simulink model "mdl3"  (R2022b)
settings: Solver=VariableStepAuto  StartTime=0.0  StopTime=3000  RelTol=1e-3
undefined symbols (not defined in the file or in its folder): DiscIntNeverNeededParam
libraries: simulink x7, rllib x1
settings Model: Creator=yonat  LastModifiedBy=yonat

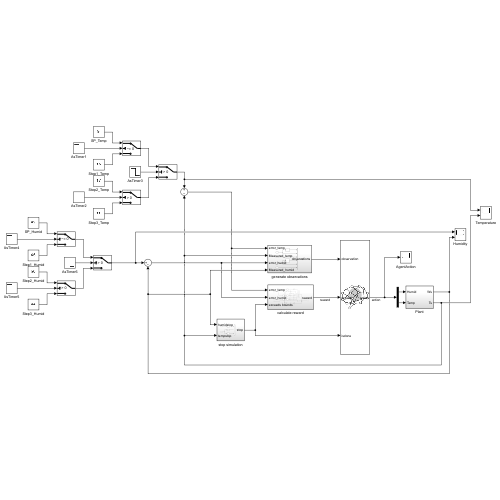
[thumbnail: Simulink's stored preview of the top-level diagram]
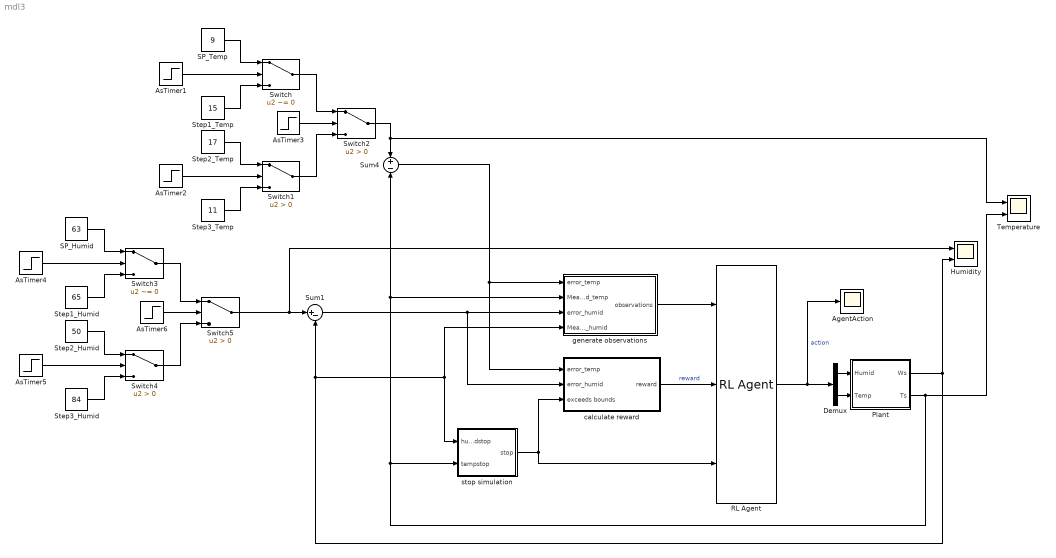
== system mdl3 ==
  AgentAction : Scope
  AsTimer1 : Step  Time=600  Before=1  After=0  SampleTime=0
  AsTimer2 : Step  Time=1800  Before=1  After=0  SampleTime=0
  AsTimer3 : Step  Time=1200  Before=1  After=0  SampleTime=0
  AsTimer4 : Step  Time=600  Before=1  After=0  SampleTime=0
  AsTimer5 : Step  Time=1800  Before=1  After=0  SampleTime=0
  AsTimer6 : Step  Time=1200  Before=1  After=0  SampleTime=0
  Demux : Demux  Outputs=2
  Humidity : Scope  NumInputPorts=2
  Plant : Subsystem
  RL Agent : rllib/RL Agent  Agent=agentObj  ExternalActionAsInput=off  ProvideLastAction=off  ProvideCumRwd=off  TreatAsDirectFeedthrough=on  UseStrictObservationDataTypes=off
  SP_Humid : Constant  Value=63
  SP_Temp : Constant  Value=9
  Step1_Humid : Constant  Value=65
  Step1_Temp : Constant  Value=15
  Step2_Humid : Constant  Value=50
  Step2_Temp : Constant  Value=17
  Step3_Humid : Constant  Value=84
  Step3_Temp : Constant  Value=11
  Sum1 : Sum  Inputs=|+-  SaturateOnIntegerOverflow=on
  Sum4 : Sum  Inputs=+-  SaturateOnIntegerOverflow=on
  Switch : Switch  Criteria=u2 ~= 0  Threshold=1  SaturateOnIntegerOverflow=off  InputSameDT=off
  Switch{1..2,4..5} (4 alike) : Switch  Criteria=u2 > Threshold  SaturateOnIntegerOverflow=off  InputSameDT=off
  Switch3 : Switch  Criteria=u2 ~= 0  Threshold=1  SaturateOnIntegerOverflow=off  InputSameDT=off
  Temperature : Scope  NumInputPorts=2
  calculate reward : Subsystem
  generate observations : Subsystem
  stop simulation : Subsystem
  wires:
  stop simulation/1(stop) -> calculate reward/3(exceeds bounds), RL Agent/3
  Plant/2(Ts) -> generate observations/2(Measured_temp), Sum4/2, stop simulation/2(tempstop), Temperature/2
  Sum4/1 -> generate observations/1(error_temp), calculate reward/1(error_temp)
  calculate reward/1(reward) -> RL Agent/2  "reward"
  Plant/1(Ws) -> generate observations/4(Measured_humid), stop simulation/1(humidstop), Sum1/2, Humidity/2
  Sum1/1 -> calculate reward/2(error_humid), generate observations/3(error_humid)
  RL Agent/1 -> AgentAction/1, Demux/1  "action"
  generate observations/1(observations) -> RL Agent/1
  Demux/2 -> Plant/2(Temp)
  Demux/1 -> Plant/1(Humid)
  SP_Temp/1 -> Switch/1
  AsTimer1/1 -> Switch/2
  Step3_Temp/1 -> Switch1/3
  Step1_Temp/1 -> Switch/3
  Switch/1 -> Switch2/1
  Switch1/1 -> Switch2/3
  AsTimer3/1 -> Switch2/2
  Step2_Temp/1 -> Switch1/1
  AsTimer2/1 -> Switch1/2
  Switch2/1 -> Temperature/1, Sum4/1
  AsTimer6/1 -> Switch5/2
  Step2_Humid/1 -> Switch4/1
  AsTimer5/1 -> Switch4/2
  Switch4/1 -> Switch5/3
  Step3_Humid/1 -> Switch4/3
  AsTimer4/1 -> Switch3/2
  Switch3/1 -> Switch5/1
  Step1_Humid/1 -> Switch3/3
  SP_Humid/1 -> Switch3/1
  Switch5/1 -> Humidity/1, Sum1/1

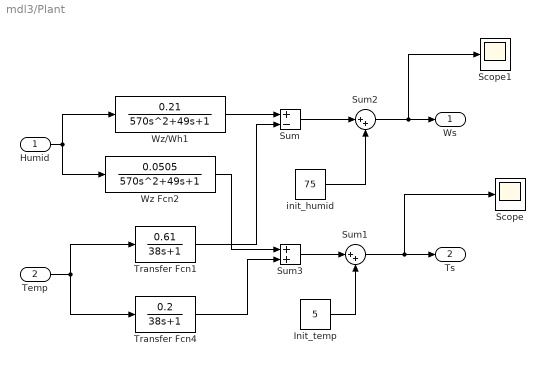
== system mdl3/Plant ==
  Humid : Inport
  Temp : Inport  Port=2
  Init_temp : Constant  Value=5
  Scope : Scope
  Scope1 : Scope
  Sum : Sum  Inputs=+-
  Sum1 : Sum  Inputs=|++
  Sum2 : Sum  Inputs=|++
  Sum3 : Sum
  Transfer Fcn1 : TransferFcn  Numerator=[0.61]  Denominator=[38 1]
  Transfer Fcn4 : TransferFcn  Numerator=[0.2]  Denominator=[38 1]
  Wz Fcn2 : TransferFcn  Numerator=[0.0505]  Denominator=[570 49 1]
  Wz/Wh1 : TransferFcn  Numerator=[0.21]  Denominator=[570 49 1]
  init_humid : Constant  Value=75
  Ws : Outport
  Ts : Outport  Port=2
  wires:
  Wz Fcn2/1 -> Sum3/1
  Humid/1 -> Wz/Wh1/1, Wz Fcn2/1
  Temp/1 -> Transfer Fcn1/1, Transfer Fcn4/1
  Transfer Fcn1/1 -> Sum/2
  Wz/Wh1/1 -> Sum/1
  Transfer Fcn4/1 -> Sum3/2
  Sum/1 -> Sum2/1
  Sum3/1 -> Sum1/1
  Sum1/1 -> Scope/1, Ts/1
  Sum2/1 -> Scope1/1, Ws/1
  Init_temp/1 -> Sum1/2
  init_humid/1 -> Sum2/2

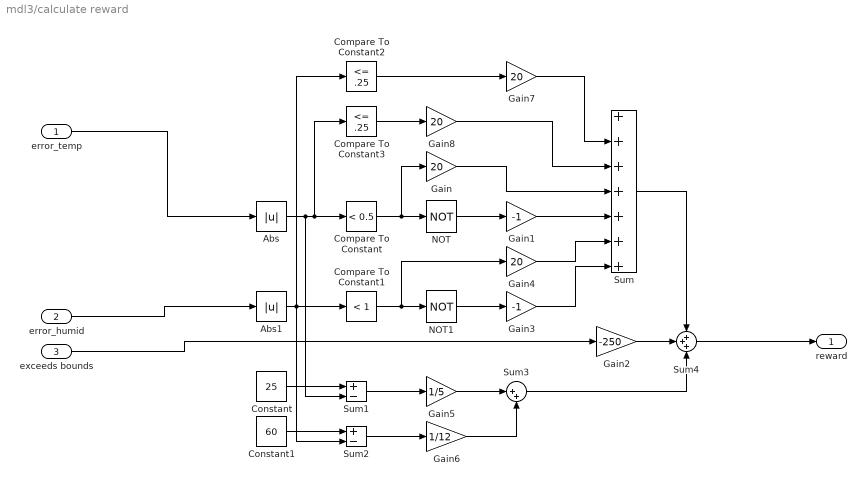
== system mdl3/calculate reward ==
  error_temp : Inport
  error_humid : Inport  Port=2
  exceeds bounds : Inport  Port=3
  Abs : Abs  SaturateOnIntegerOverflow=off
  Abs1 : Abs  SaturateOnIntegerOverflow=off
  Compare To Constant : simulink/Logic and Bit Operations/Compare To Constant  relop=<  const=0.5  OutDataTypeStr=boolean
  Compare To Constant1 : simulink/Logic and Bit Operations/Compare To Constant  relop=<  const=1  OutDataTypeStr=boolean
  Compare To Constant2 : simulink/Logic and Bit Operations/Compare To Constant  relop=<=  const=.25  OutDataTypeStr=boolean
  Compare To Constant3 : simulink/Logic and Bit Operations/Compare To Constant  relop=<=  const=.25  OutDataTypeStr=boolean
  Constant : Constant  Value=25
  Constant1 : Constant  Value=60
  Gain{,4,7..8} (4 alike) : Gain  Gain=20
  Gain1 : Gain  Gain=-1
  Gain2 : Gain  Gain=-250
  Gain3 : Gain  Gain=-1
  Gain5 : Gain  Gain=1/5
  Gain6 : Gain  Gain=1/12
  NOT : Logic  Operator=NOT  IconShape=distinctive  AllPortsSameDT=off  OutDataTypeStr=boolean
  NOT1 : Logic  Operator=NOT  IconShape=distinctive  AllPortsSameDT=off  OutDataTypeStr=boolean
  Sum : Sum  Inputs=+++++++  OutDataTypeStr=double
  Sum1 : Sum  Inputs=+-
  Sum2 : Sum  Inputs=+-
  Sum3 : Sum  Inputs=|++
  Sum4 : Sum  Inputs=+++
  reward : Outport  VectorParamsAs1DForOutWhenUnconnected=off
  wires:
  Compare To Constant2/1 -> Gain7/1
  Abs1/1 -> Compare To Constant1/1, Compare To Constant2/1, Sum2/2
  Sum3/1 -> Sum4/3
  NOT/1 -> Gain1/1
  Sum4/1 -> reward/1
  Gain7/1 -> Sum/2
  NOT1/1 -> Gain3/1
  Gain6/1 -> Sum3/2
  Sum2/1 -> Gain6/1
  Sum1/1 -> Gain5/1
  exceeds bounds/1 -> Gain2/1
  Compare To Constant1/1 -> Gain4/1, NOT1/1
  Gain/1 -> Sum/4
  Constant/1 -> Sum1/1
  Gain5/1 -> Sum3/1
  error_temp/1 -> Abs/1
  Compare To Constant/1 -> NOT/1, Gain/1
  Abs/1 -> Compare To Constant3/1, Compare To Constant/1, Sum1/2
  Sum/1 -> Sum4/1
  Gain2/1 -> Sum4/2
  Gain8/1 -> Sum/3
  Gain3/1 -> Sum/7
  Compare To Constant3/1 -> Gain8/1
  error_humid/1 -> Abs1/1
  Gain1/1 -> Sum/5
  Gain4/1 -> Sum/6
  Constant1/1 -> Sum2/1

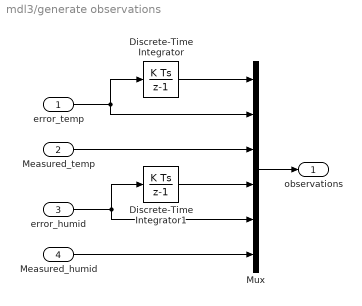
== system mdl3/generate observations ==
  error_temp : Inport
  Measured_temp : Inport  Port=2
  error_humid : Inport  Port=3
  Measured_humid : Inport  Port=4
  Discrete-Time Integrator : DiscreteIntegrator  SampleTime=1.0  ICPrevOutput=DiscIntNeverNeededParam  ICPrevScaledInput=DiscIntNeverNeededParam
  Discrete-Time Integrator1 : DiscreteIntegrator  SampleTime=1.0  ICPrevOutput=DiscIntNeverNeededParam  ICPrevScaledInput=DiscIntNeverNeededParam
  Mux : Mux  Inputs=6
  observations : Outport  VectorParamsAs1DForOutWhenUnconnected=off
  wires:
  error_temp/1 -> Discrete-Time Integrator/1, Mux/2
  error_humid/1 -> Mux/5, Discrete-Time Integrator1/1
  Discrete-Time Integrator1/1 -> Mux/4
  Discrete-Time Integrator/1 -> Mux/1
  Measured_temp/1 -> Mux/3
  Measured_humid/1 -> Mux/6
  Mux/1 -> observations/1

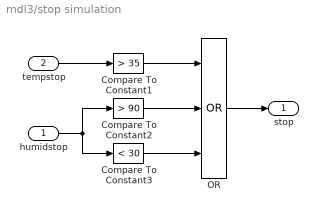
== system mdl3/stop simulation ==
  humidstop : Inport
  tempstop : Inport  Port=2
  Compare To Constant1 : simulink/Logic and Bit Operations/Compare To Constant  relop=>  const=35  OutDataTypeStr=boolean
  Compare To Constant2 : simulink/Logic and Bit Operations/Compare To Constant  relop=>  const=90  OutDataTypeStr=boolean
  Compare To Constant3 : simulink/Logic and Bit Operations/Compare To Constant  relop=<  const=30  OutDataTypeStr=boolean
  OR : Logic  Operator=OR  Inputs=3  IconShape=distinctive  AllPortsSameDT=off  OutDataTypeStr=boolean
  stop : Outport  VectorParamsAs1DForOutWhenUnconnected=off
  wires:
  tempstop/1 -> Compare To Constant1/1
  humidstop/1 -> Compare To Constant2/1, Compare To Constant3/1
  Compare To Constant1/1 -> OR/1
  Compare To Constant3/1 -> OR/3
  OR/1 -> stop/1
  Compare To Constant2/1 -> OR/2
